simulink model "GenerateTriggerSignal"  (R2016b)
settings: Solver=FixedStepDiscrete  StartTime=0.0  StopTime=inf  FixedStep=sCoreParams.core.stepPeriod  RelTol=1e-3  EnableMultiTasking=on
undefined symbols (not defined in the file): sCoreParams, sCoreParams_decoders_txDetector_stimTriggerChannel, sCoreParams_decoders_txDetector_triggerChannel
libraries: dspsrcs4 x3, dspswit3 x2, dspindex x2
settings Model: DataTypeOverride=Double  MinMaxOverflowLogging=ForceOff  Creator=rzelmann  LastModifiedBy=rzelmann
settings SolverCC: EnableConcurrentExecution=on  AutoInsertRateTranBlk=on
settings DataIOCC: SaveFormat=StructureWithTime
settings OptimizationCC: BlockReduction=off  DefaultParameterBehavior=Inlined  OptimizeBlockIOStorage=off  BufferReuse=off  GlobalBufferReuse=off  ExpressionFolding=off  LocalBlockOutputs=off  LifeSpan=inf
settings DebuggingCC: SFUnexpectedBacktrackingDiag=warning  SFNoUnconditionalDefaultTransitionDiag=warning  SFExecutionAtInitializationDiag=none
settings HardwareCC: ProdBitPerPointer=32  ProdBitPerSizeT=32  ProdBitPerPtrDiffT=32  ProdLargestAtomicFloat=None  ProdWordSize=32  ProdLongLongMode=on  ProdHWDeviceType=Generic->32-bit x86 compatible
settings ModelReferenceCC: EnableParallelModelReferenceBuilds=on  ParallelModelReferenceMATLABWorkerInit=Copy Base Workspace  ModelReferenceNumInstancesAllowed=Single  ModelReferencePassRootInputsByReference=off
settings RTWCC: SystemTargetFile=slrt.tlc  TemplateMakefile=slrt_default_tmf  Description=Simulink Real-Time  RTWCompilerOptimization=on
settings CodeAppCC: MaxIdLength=63
settings ConfigComp: CovMetricSettings=dw  CovHtmlReporting=on  CovSaveCumulativeToWorkspaceVar=on  CovSaveSingleToWorkspaceVar=on  CovExternalEMLEnable=off

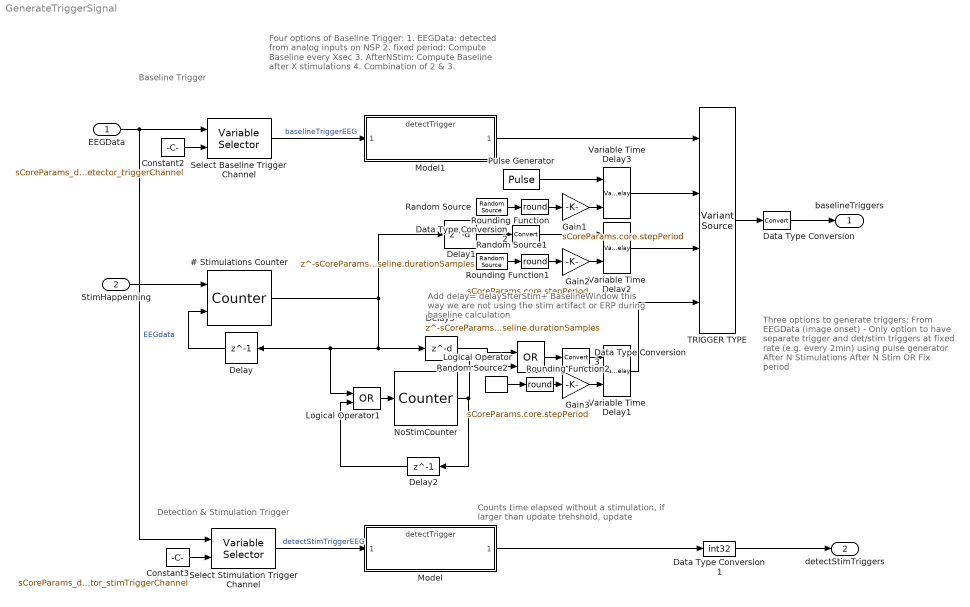
== system GenerateTriggerSignal ==
  note: Four options of Baseline Trigger:
      | 1. EEGData: detected from analog inputs on NSP
      | 2. fixed period: Compute Baseline every Xsec
      | 3. AfterNStim: Compute Baseline after X stimulations
      | 4. Combination of 2 & 3.
  note: Add delay= delaySfterStim+ BaselineWindow
      | this way we are not using the stim artifact or ERP
      | during baseline calculation
  note: Counts time elapsed without a stimulation,
      | if larger than update trehshold, update
  note: Three options to generate triggers:
      | From EEGData (image onset)
      | - Only option to have separate
      | trigger and det/stim triggers
      | at fixed rate (e.g. every 2min)
      | using pulse generator
      | After N Stimulations
      | After N Stim OR Fix period
  note: Detection & Stimulation Trigger
  note: Baseline Trigger
  EEGData : Inport  OutDataTypeStr=double  PortDimensions=[sCoreParams.core.samplesPerStep sCoreParams.core.maxChannelsPerNSP]  SampleTime=sCoreParams.core.stepPeriod
  StimHappenning : Inport  Port=2  OutDataTypeStr=boolean  SampleTime=sCoreParams.core.stepPeriod
  # Stimulations Counter : dspswit3/Counter  Direction=Up  CountEvent=Rising edge  CounterSize=User defined  MaxCount=255  InitialCount=0  Output=Hit  HitValue=sCoreParams.triggers.numStimulations  ResetInput=on  SamplesPerFrame=1  Ts=1  CntDtype=double  HitDtype=Logical
  Constant2 : Constant  Value=sCoreParams_decoders_txDetector_triggerChannel
  Constant3 : Constant  Value=sCoreParams_decoders_txDetector_stimTriggerChannel
  Data Type Conversion : DataTypeConversion
  Data Type Conversion1 : DataTypeConversion  OutDataTypeStr=int32
  Data Type Conversion2 : DataTypeConversion
  Data Type Conversion3 : DataTypeConversion
  Delay : Delay  DelayLength=1
  Delay1 : Delay  DelayLength=sCoreParams.decoders.txDetector.delayAfterStimSamples+sCoreParams.Features.Baseline.durationSamples
  Delay2 : Delay  DelayLength=1  InitialCondition=1
  Delay3 : Delay  DelayLength=sCoreParams.decoders.txDetector.delayAfterStimSamples+sCoreParams.Features.Baseline.durationSamples
  Gain1 : Gain  Gain=sCoreParams.core.stepPeriod
  Gain2 : Gain  Gain=sCoreParams.core.stepPeriod
  Gain3 : Gain  Gain=sCoreParams.core.stepPeriod
  Logical Operator : Logic  Operator=OR  IconShape=distinctive  AllPortsSameDT=off  OutDataTypeStr=boolean
  Logical Operator1 : Logic  Operator=OR  IconShape=distinctive  AllPortsSameDT=off  OutDataTypeStr=boolean
  Model : ModelReference  ModelNameDialog=detectTrigger.slx  SimulationMode=Normal  ModelReferenceVersion=1.17
  Model1 : ModelReference  ModelNameDialog=detectTrigger.slx  SimulationMode=Normal  ModelReferenceVersion=1.17
  NoStimCounter : dspswit3/Counter  Direction=Up  CountEvent=Free running  CounterSize=User defined  MaxCount=sCoreParams.triggers.periodSamples*2  InitialCount=0  Output=Hit  HitValue=sCoreParams.triggers.periodSamples  ResetInput=on  SamplesPerFrame=1  Ts=sCoreParams.core.stepPeriod  CntDtype=double  HitDtype=Logical
  Pulse Generator : DiscretePulseGenerator  Period=sCoreParams.triggers.periodSamples  PhaseDelay=min(sCoreParams.triggers.initialTriggerSamples, sCoreParams.triggers.periodSamples-1)  SampleTime=sCoreParams.core.stepPeriod  VectorParams1D=off
  Random Source : dspsrcs4/Random Source  SrcType=Uniform  NormMethod=Ziggurat  CltLength=12  MinVal=0  MaxVal=sCoreParams.triggers.periodJitterInteger  MeanVal=0  VarVal=1  RepMode=Not repeatable  rawSeed=1  IsInherit=off  SampMode=Discrete  SampTime=sCoreParams.core.stepPeriod  SampFrame=1  DataType=Double  OutComplex=Real  OutputFrames=off
  Random Source1 : dspsrcs4/Random Source  SrcType=Uniform  NormMethod=Ziggurat  CltLength=12  MinVal=0  MaxVal=sCoreParams.triggers.periodJitterInteger  MeanVal=0  VarVal=1  RepMode=Not repeatable  rawSeed=1  IsInherit=off  SampMode=Discrete  SampTime=sCoreParams.core.stepPeriod  SampFrame=1  DataType=Double  OutComplex=Real  OutputFrames=off
  Random Source2 : dspsrcs4/Random Source  SrcType=Uniform  NormMethod=Ziggurat  CltLength=12  MinVal=0  MaxVal=sCoreParams.triggers.periodJitterInteger  MeanVal=0  VarVal=1  RepMode=Not repeatable  rawSeed=1  IsInherit=off  SampMode=Discrete  SampTime=sCoreParams.core.stepPeriod  SampFrame=1  DataType=Double  OutComplex=Real  OutputFrames=off
  Rounding Function : Rounding  Operator=round
  Rounding Function1 : Rounding  Operator=round
  Rounding Function2 : Rounding  Operator=round
  Select Baseline Trigger Channel : dspindex/Variable Selector  NumInputs=1  rowsOrCols=Columns  IdxMode=Variable  Elements=sCoreParams_decoders_txDetector_triggerChannel  ZerOneIdxMode=One-based  errmode=Clip Index  FillMode=on  FillValues=0
  Select Stimulation Trigger Channel : dspindex/Variable Selector  NumInputs=1  rowsOrCols=Columns  IdxMode=Variable  Elements=sCoreParams_decoders_txDetector_triggerChannel  ZerOneIdxMode=One-based  errmode=Clip Index  FillMode=on  FillValues=0
  TRIGGER TYPE : VariantSource
  Variable Time Delay1 : VariableTransportDelay  MaximumDelay=sCoreParams.core.stepPeriod*sCoreParams.triggers.periodJitterInteger  MaximumPoints=sCoreParams.core.samplesPerStep*sCoreParams.triggers.periodJitterInteger+1  ZeroDelay=on  TransDelayFeedthrough=on
  Variable Time Delay2 : VariableTransportDelay  MaximumDelay=sCoreParams.core.stepPeriod*sCoreParams.triggers.periodJitterInteger  MaximumPoints=sCoreParams.core.samplesPerStep*sCoreParams.triggers.periodJitterInteger+1  ZeroDelay=on  TransDelayFeedthrough=on
  Variable Time Delay3 : VariableTransportDelay  MaximumDelay=sCoreParams.core.stepPeriod*sCoreParams.triggers.periodJitterInteger  MaximumPoints=sCoreParams.core.samplesPerStep*sCoreParams.triggers.periodJitterInteger+1  FixedBuffer=on  ZeroDelay=on
  baselineTriggers : Outport  OutDataTypeStr=int32
  detectStimTriggers : Outport  Port=2  OutDataTypeStr=int32  SampleTime=sCoreParams.core.stepPeriod
  wires:
  # Stimulations Counter/1 -> Logical Operator1/1, Delay/1, Delay3/1, Delay1/1
  Delay/1 -> # Stimulations Counter/2
  Variable Time Delay2/1 -> TRIGGER TYPE/3
  StimHappenning/1 -> # Stimulations Counter/1
  TRIGGER TYPE/1 -> Data Type Conversion/1
  Constant2/1 -> Select Baseline Trigger Channel/2
  Select Baseline Trigger Channel/1 -> Model1/1  "baselineTriggerEEG"
  Model1/1 -> TRIGGER TYPE/1
  Variable Time Delay3/1 -> TRIGGER TYPE/2
  Variable Time Delay1/1 -> TRIGGER TYPE/4
  EEGData/1 -> Select Stimulation Trigger Channel/1, Select Baseline Trigger Channel/1  "EEGdata"
  Constant3/1 -> Select Stimulation Trigger Channel/2
  Select Stimulation Trigger Channel/1 -> Model/1  "detectStimTriggerEEG"
  Model/1 -> Data Type Conversion1/1
  Gain1/1 -> Variable Time Delay3/2
  Pulse Generator/1 -> Variable Time Delay3/1
  Random Source1/1 -> Rounding Function1/1
  Gain2/1 -> Variable Time Delay2/2
  Delay1/1 -> Data Type Conversion2/1
  Random Source2/1 -> Rounding Function2/1
  Gain3/1 -> Variable Time Delay1/2
  NoStimCounter/1 -> Delay2/1, Logical Operator/2
  Data Type Conversion/1 -> baselineTriggers/1
  Data Type Conversion1/1 -> detectStimTriggers/1
  Data Type Conversion2/1 -> Variable Time Delay2/1
  Logical Operator/1 -> Data Type Conversion3/1
  Data Type Conversion3/1 -> Variable Time Delay1/1
  Random Source/1 -> Rounding Function/1
  Rounding Function/1 -> Gain1/1
  Rounding Function1/1 -> Gain2/1
  Rounding Function2/1 -> Gain3/1
  Logical Operator1/1 -> NoStimCounter/1
  Delay2/1 -> Logical Operator1/2
  Delay3/1 -> Logical Operator/1
